simulink model "sedemo_shared_proc"  (Simulink 7.5)
settings: Solver=VariableStepDiscrete  StartTime=0.0  StopTime=40  MaxStep=inf  RelTol=1e-3
undefined symbols (not defined in the file or in its folder): des_attributefunction_support
libraries: simeventssink1 x7, simeventsattributes2 x4, simeventsgenerators1 x3, simeventsrouting1 x3, simeventsserver1 x2, simeventsqueue1 x2, simeventsinfo x1, simeventstranslate1 x1
settings Model: Creator=The MathWorks Inc.  ExtModeAutoUpdateStatusClock=off
settings DataIOCC: SaveOutput=off  SignalLogging=off  SaveTime=off
settings OptimizationCC: InitFltsAndDblsToZero=on
settings DebuggingCC: AlgebraicLoopMsg=error  SignalResolutionControl=TryResolveAllWithWarning  SolverPrmCheckMsg=none  StrictBusMsg=Warning
settings SimEventsCC: propDiagAttribOutput=1  propDiagFcnCallOutput=1  propDiagStatOutput=0

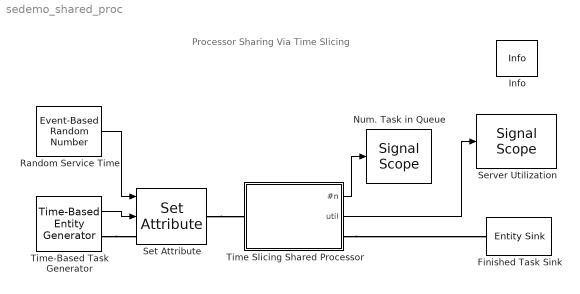
== system sedemo_shared_proc ==
  note: Processor Sharing Via Time Slicing
  Finished Task Sink : simeventssink1/Entity Sink  Priority=1  SystemSampleTime=-1  AvailableForArrivals=on  StatNumberArrived=Off
  Info : simeventsinfo/Info  SystemSampleTime=-1
  Num. Task in Queue : simeventssink1/Signal Scope  Priority=1  SystemSampleTime=-1  PlotType=Stair  InputType=Signal  NumInputs=1  AttributeNameY=Count  XInputOptionSignal=Event time  XInputOptionEntity=Event time  AttributeNameX=Count  EnableEntityOutport=on  XMin=-0.4  XMax=40.4  XLimitExceededOption=Stretch axis limits  YLimitExceededOption=Stretch axis limits  AxisGrid=on  AxisLegend=off  LineDisables=""  LineColors=b  LineStyles=-  LineMarkers=.  OpenScopeAtSimStart=on  Title=Number in Shared Processor Queue  YLabel=Number  XLabel=Time  FigurePosition=[324 514 300 188]  AxisZoom=off  DataStoreOption=Limited  DataPointsLimit=100000  StatNumberArrived=Off  ShowCountPlotted=off  ShowToolbar=off
      settings: YMin=-0.04  YMax=4.04
  Random Service Time : simeventsgenerators1/Signal Generators/Event-Based Random Number  SystemSampleTime=-1  distribution=Exponential  meanExp=1/3  minUnif=1  maxUnif=1  pOneBern=0.25  pSuccessBino=0.5  numTrialBino=1  meanNorm=0  stdNorm=1  minTri=1  maxTri=3  modeTri=2  thresholdLogn=0  scaleLogn=1  shapeLogn=1  pSuccessGeo=0.5  meanPoiss=1  thresholdLogl=0  scaleLogl=1  thresholdGam=0  scaleGam=1  shapeGam=1  minBeta=0  maxBeta=1  shape1Beta=1  shape2Beta=1  minUnid=0  maxUnid=1  numValueUnid=2  thresholdWbl=0  scaleWbl=1  shapeWbl=1  valueVecCont=[0 1]  cdfVecCont=[0 1]  valueVecDisc=[0 1]  probVecDisc=[0.5 0.5]  seed=12345  IsProcessed=on  isConnected=1
  Server Utilization : simeventssink1/Signal Scope  Priority=1  SystemSampleTime=-1  PlotType=Stair  InputType=Signal  NumInputs=1  AttributeNameY=Count  XInputOptionSignal=Event time  XInputOptionEntity=Event time  AttributeNameX=Count  EnableEntityOutport=on  XMin=-0.4  XMax=40.4  XLimitExceededOption=Stretch axis limits  YLimitExceededOption=Stretch axis limits  AxisGrid=on  AxisLegend=off  LineDisables=""  LineColors=b  LineStyles=-  LineMarkers=.  OpenScopeAtSimStart=on  Title=Shared Processor Utilization  YLabel=Utilization  XLabel=Time  FigurePosition=[324 288 299 178]  AxisZoom=off  DataStoreOption=Limited  DataPointsLimit=10000  StatNumberArrived=Off  ShowCountPlotted=off  ShowToolbar=off
      settings: YMin=-0.01  YMax=1.01
  Set Attribute : simeventsattributes2/Set Attribute  Priority=1  DialogController=des_ddg_create  DialogControllerArgs=DataTag4  SystemSampleTime=-1  AttributeFrom=Dialog|Signal port|Signal port  AttributeName=Priority|TaskExecTime|JobNumber  AttributeTreatAsVector=1|1|1  AttributeValue=2|1|1  AttributeCreate=on  StatNumberDeparted=Off  EvaluatedAttributeValue={2;[];[]}
  Time Slicing Shared Processor : Subsystem
  Time-Based Task Generator : simeventsgenerators1/Entity Generators/Time-Based Entity Generator  Priority=1  DialogController=des_ddg_create  DialogControllerArgs=DataTag26  SystemSampleTime=-1  GenerateEntitiesUpon=Intergeneration time from dialog  Distribution=Exponential  Minimum=0  Maximum=1  Mean=1/2  InitialSeed=54321  Period=1  PriorityEntityGeneration=300  GenerateEntityAtSimulationStart=off  ResponseWhenBlocked=Pause generation  ResponseWhenUnblocked=Immediate restart  EntityType=Standard  StatNumberDeparted=On  StatPendingEntity=Off  StatAverageIntergenerationTime=Off
  wires:
  Random Service Time/1 -> Set Attribute/1
  Time Slicing Shared Processor/2(util) -> Server Utilization/1
  Time-Based Task Generator/1 -> Set Attribute/2
  Time Slicing Shared Processor/1(#n) -> Num. Task in Queue/1
  connections:
  Time-Based Task Generator/RConn1 -- Set Attribute/LConn1
  Time Slicing Shared Processor/RConn1 -- Finished Task Sink/LConn1
  Set Attribute/RConn1 -- Time Slicing Shared Processor/LConn1

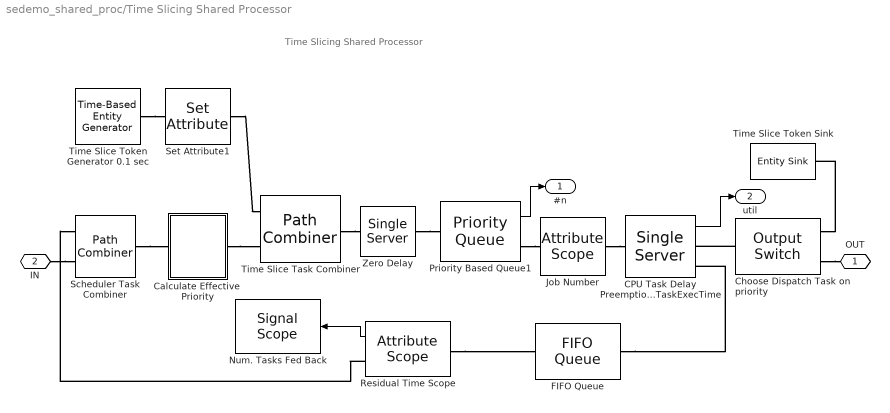
== system sedemo_shared_proc/Time Slicing Shared Processor ==
  note: Time Slicing Shared Processor
  CPU Task Delay Preemption on priority Residual TaskExecTime : simeventsserver1/Single Server  Priority=1  SystemSampleTime=-1  ServiceTimeFrom=Attribute  ServiceTime=0.5  AttributeName=TaskExecTime  PriorityServiceCompletion=4  PermitPreemption=on  SortingAttributeName=EffectivePriority  SortingDirection=Ascending  WriteToAttribute=on  ResidualAttributeName=TaskExecTime  CreateAttribute=off  EnableTOPort=off  StatNumberDeparted=Off  StatNumberInBlock=Off  StatNumberPreempted=Off  StatPendingEntity=Off  StatAverageWait=Off  StatUtilization=On  StatNumberTimedout=Off
  Calculate Effective  Priority : Subsystem  LoadFcn=des_attributefunction_support(gcb,'LoadFcn');  StartFcn=des_attributefunction_support(gcb,'StartFcn');  mask(Attribute Function){OutputNamePrefix=out_}
      mask prompts: OutputNamePrefix "Prefix name"
      settings: CopyFcn=des_attributefunction_support(gcb,'CopyFcn');  OpenFcn=des_attributefunction_support(gcb,'OpenFcn');  ErrorFcn=des_error_redirect
      mask Display: image(des_iconLoad('attribFunction.jpg'),'center');
  Choose Dispatch Task on priority : simeventsrouting1/Output Switch  Priority=1  SystemSampleTime=-1  NumberOutputPorts=2  SwitchingCriterion=From attribute  InitialSeed=34567  AttributeName=Priority  InitialConditionsOpt=off  InitialConditions=1  EntityBufferOpt=off  SpecifyEventPriority=off  PriorityOutputSwitchSelectPort=4100  TimeoutPortOpt=off  StatNumberDeparted=Off  StatNumberTimedOut=Off  StatPendingEntity=Off  StatLastDeparturePort=Off  EvaluatedNumPorts=2
  FIFO Queue : simeventsqueue1/FIFO Queue  Priority=1  SystemSampleTime=-1  Capacity=inf  EnableTOPort=off  StatNumberDeparted=Off  StatNumberInBlock=Off  StatPendingEntity=Off  StatAverageWait=Off  StatAverageQueueLength=Off  StatNumberTimedout=Off
  Job Number : simeventssink1/Attribute Scope  Priority=1  SystemSampleTime=-1  PlotType=Stair  InputType=Attribute  NumInputs=1  AttributeNameY=JobNumber  XInputOptionSignal=Event time  XInputOptionEntity=Event time  AttributeNameX=Count  EnableEntityOutport=on  XMin=-0.4  XMax=40.4  XLimitExceededOption=Stretch axis limits  YLimitExceededOption=Stretch axis limits  AxisGrid=on  AxisLegend=off  LineDisables=""  LineColors=b  LineStyles=None  LineMarkers=.  OpenScopeAtSimStart=on  Title=Jobs in Shared Processor  YLabel=Job Number (ID)  XLabel=Time  FigurePosition=[11 288 301 179]  AxisZoom=off  DataStoreOption=Limited  DataPointsLimit=10000  StatNumberArrived=Off  ShowCountPlotted=off  ShowToolbar=off
      settings: YMin=-1.74  YMax=73.74
  Num. Tasks Fed Back : simeventssink1/Signal Scope  Priority=1  SystemSampleTime=-1  PlotType=Stair  InputType=Signal  NumInputs=1  AttributeNameY=Count  XInputOptionSignal=Event time  XInputOptionEntity=Event time  AttributeNameX=Count  EnableEntityOutport=on  XMin=0  XMax=10  XLimitExceededOption=Stretch axis limits  YLimitExceededOption=Stretch axis limits  AxisGrid=on  AxisLegend=off  LineDisables=""  LineColors=b  LineStyles=-  LineMarkers=.  OpenScopeAtSimStart=off  Title="# of Tasks  Fed Back"  YLabel=""  XLabel=Time  FigurePosition=[93 743 321 192]  AxisZoom=off  DataStoreOption=Limited  DataPointsLimit=10000  StatNumberArrived=Off  ShowCountPlotted=off  ShowToolbar=off
      settings: YMin=0  YMax=10
  Priority Based Queue1 : simeventsqueue1/Priority Queue  Priority=1  SystemSampleTime=-1  Capacity=128  SortingAttributeName=EffectivePriority  SortingDirection=Ascending  EnableTOPort=off  StatNumberDeparted=Off  StatNumberInBlock=On  StatPendingEntity=Off  StatAverageWait=Off  StatAverageQueueLength=Off  StatNumberTimedout=Off
  Residual Time Scope : simeventssink1/Attribute Scope  Priority=1  SystemSampleTime=-1  PlotType=Stair  InputType=Attribute  NumInputs=1  AttributeNameY=TaskExecTime  XInputOptionSignal=Event time  XInputOptionEntity=Event time  AttributeNameX=Count  EnableEntityOutport=on  XMin=0  XMax=40  XLimitExceededOption=Stretch axis limits  YLimitExceededOption=Stretch axis limits  AxisGrid=on  AxisLegend=off  LineDisables=""  LineColors=b  LineStyles=None  LineMarkers=.  OpenScopeAtSimStart=on  Title=Residual Service Time for Tasks  YLabel=Residual Time  XLabel=Time  FigurePosition=[12 515 301 186]  AxisZoom=off  DataStoreOption=Limited  DataPointsLimit=10000  StatNumberArrived=On  ShowCountPlotted=off  ShowToolbar=off
      settings: YMin=0  YMax=2
  Scheduler Task Combiner : simeventsrouting1/Path Combiner  Priority=1  SystemSampleTime=-1  NumberInputPorts=2  InputPortPrecedence=IN1 port  InitialSeed=45675  SpecifyEventPriority=off  PriorityPathCombinerPortPrecedenceSelection=4100  StatNumberDeparted=Off  StatLastArrivalPort=Off  EvaluatedNumPorts=2
  Set Attribute1 : simeventsattributes2/Set Attribute  Priority=1  DialogController=des_ddg_create  DialogControllerArgs=DataTag19  SystemSampleTime=-1  AttributeFrom=Dialog|Dialog|Dialog|Dialog  AttributeName=Priority|TaskExecTime|JobNumber|EffectivePriority  AttributeTreatAsVector=1|1|1|1  AttributeValue=1|0|-1|1  AttributeCreate=on  StatNumberDeparted=Off  EvaluatedAttributeValue={1}
  Time Slice Token Generator 0.1 sec : simeventsgenerators1/Entity Generators/Time-Based Entity Generator  Priority=1  DialogController=des_ddg_create  DialogControllerArgs=DataTag21  SystemSampleTime=-1  GenerateEntitiesUpon=Intergeneration time from dialog  Distribution=Constant  Minimum=0  Maximum=1  Mean=1  InitialSeed=12345  Period=.1  PriorityEntityGeneration=10  GenerateEntityAtSimulationStart=on  ResponseWhenBlocked=Pause generation  ResponseWhenUnblocked=Immediate restart  EntityType=Standard  StatNumberDeparted=Off  StatPendingEntity=Off  StatAverageIntergenerationTime=Off
  Time Slice Token Sink : simeventssink1/Entity Sink  Priority=1  SystemSampleTime=-1  AvailableForArrivals=on  StatNumberArrived=Off
  Time Slice Task Combiner : simeventsrouting1/Path Combiner  Priority=1  SystemSampleTime=-1  NumberInputPorts=2  InputPortPrecedence=IN1 port  InitialSeed=45675  SpecifyEventPriority=off  PriorityPathCombinerPortPrecedenceSelection=4100  StatNumberDeparted=Off  StatLastArrivalPort=Off  EvaluatedNumPorts=2
  Zero Delay : simeventsserver1/Single Server  Priority=1  SystemSampleTime=-1  ServiceTimeFrom=Dialog  ServiceTime=0  AttributeName=TaskExecTime  PriorityServiceCompletion=1  PermitPreemption=off  SortingAttributeName=EffectivePriority  SortingDirection=Ascending  WriteToAttribute=off  ResidualAttributeName=TaskExecTime  CreateAttribute=off  EnableTOPort=off  StatNumberDeparted=Off  StatNumberInBlock=Off  StatNumberPreempted=Off  StatPendingEntity=Off  StatAverageWait=Off  StatUtilization=Off  StatNumberTimedout=Off
  OUT : PMIOPort  Port=1  Side=Right
  IN : PMIOPort  Port=2  Side=Left
  #n : Outport  OutDataType=sfix(16)  OutScaling=2^0
  util : Outport  Port=2  OutDataType=sfix(16)  OutScaling=2^0
  wires:
  Residual Time Scope/1 -> Num. Tasks Fed Back/1
  Priority Based Queue1/1 -> #n/1
  CPU Task Delay Preemption on priority Residual TaskExecTime/1 -> util/1
  connections:
  Job Number/RConn1 -- CPU Task Delay Preemption on priority Residual TaskExecTime/LConn1
  FIFO Queue/LConn1 -- CPU Task Delay Preemption on priority Residual TaskExecTime/RConn2
  Scheduler Task Combiner/RConn1 -- Calculate Effective  Priority/LConn1
  Calculate Effective  Priority/RConn1 -- Time Slice Task Combiner/LConn2
  Residual Time Scope/LConn1 -- FIFO Queue/RConn1
  Priority Based Queue1/RConn1 -- Job Number/LConn1
  Residual Time Scope/RConn1 -- Scheduler Task Combiner/LConn1
  Time Slice Token Generator 0.1 sec/RConn1 -- Set Attribute1/LConn1
  Set Attribute1/RConn1 -- Time Slice Task Combiner/LConn1
  IN/RConn1 -- Scheduler Task Combiner/LConn2
  Choose Dispatch Task on priority/RConn1 -- Time Slice Token Sink/LConn1
  Choose Dispatch Task on priority/LConn1 -- CPU Task Delay Preemption on priority Residual TaskExecTime/RConn1
  Choose Dispatch Task on priority/RConn2 -- OUT/RConn1
  Time Slice Task Combiner/RConn1 -- Zero Delay/LConn1
  Zero Delay/RConn1 -- Priority Based Queue1/LConn1

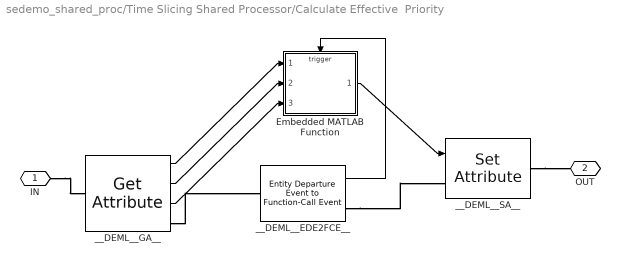
== system sedemo_shared_proc/Time Slicing Shared Processor/Calculate Effective  Priority ==
  Embedded MATLAB Function : Stateflow chart  TreatAsAtomicUnit=on
      settings: PropExecContextOutsideSubsystem=on
  __DEML__EDE2FCE__ : simeventstranslate1/Entity Departure Event to Function-Call Event  Priority=1  SystemSampleTime=-1  TimingFunctionCallF1=Before entity departure  EnableE1Port=off  EnableF2Port=off  TimingFunctionCallF2=Before entity departure  EnableE2Port=off  StatNumberDeparted=Off  StatNumberF1Calls=Off  StatNumberF2Calls=Off  IsInsideAFB=on
  __DEML__GA__ : simeventsattributes2/Get Attribute  Priority=1  DialogController=des_ddg_create  DialogControllerArgs=DataTag8  SystemSampleTime=-1  AttributeName=TaskExecTime|JobNumber|Priority  AttributeMissing=Error|Error|Error  AttributeDefaultValue=1|1|1  AttributeSendTiming=Before entity departure|Before entity departure|Before entity departure  AttributeTreatAsVector=1|1|1  StatNumberDeparted=Off  EvaluatedDefaultAttributeValue={[];[];[]}
  __DEML__SA__ : simeventsattributes2/Set Attribute  Priority=1  DialogController=des_ddg_create  DialogControllerArgs=DataTag10  SystemSampleTime=-1  AttributeFrom=Signal port  AttributeName=EffectivePriority  AttributeTreatAsVector=1  AttributeValue=1  AttributeCreate=on  StatNumberDeparted=Off  EvaluatedAttributeValue={[]}
  IN : PMIOPort  Port=1  Side=Left
  OUT : PMIOPort  Port=2  Side=Right
  wires:
  __DEML__EDE2FCE__/1 -> Embedded MATLAB Function/Trigger
  __DEML__GA__/1 -> Embedded MATLAB Function/1(TaskExecTime)
  __DEML__GA__/2 -> Embedded MATLAB Function/2(JobNumber)
  __DEML__GA__/3 -> Embedded MATLAB Function/3(Priority)
  Embedded MATLAB Function/1(out_EffectivePriority) -> __DEML__SA__/1
  connections:
  __DEML__SA__/RConn1 -- OUT/RConn1
  IN/RConn1 -- __DEML__GA__/LConn1
  __DEML__GA__/RConn1 -- __DEML__EDE2FCE__/LConn1
  __DEML__EDE2FCE__/RConn1 -- __DEML__SA__/LConn1

== matlab function Time Slicing Shared Processor/Calculate Effective Priority/Embedded MATLAB Function ==
  data: TaskExecTime input double; out_EffectivePriority output double; JobNumber input double; Priority input double
  events: trigger input FUNCTION_CALL_EVENT
function out_EffectivePriority  = ...
	fcn(TaskExecTime, JobNumber, Priority)
%FCN    Access and modify attributes with Embedded MATLAB Function 
% 
% Calculate the EffectivePriority attribute to allow for sorting by 
% TaskExecTime, JobNumber and Priority. 
%

out_EffectivePriority =  TaskExecTime -  ...
						 JobNumber * 0.001 - ...
						 Priority * 0.000001 + 1000000;
